simulink library "lib_astrodynamics"  (Simulink 7.7)
settings: Solver=ode45  StartTime=0.0  StopTime=10.0  RelTol=1e-3
libraries: lib_astrodynamics x4
settings Model: Creator=kkamiya  LastModifiedBy=yamaurashusaku

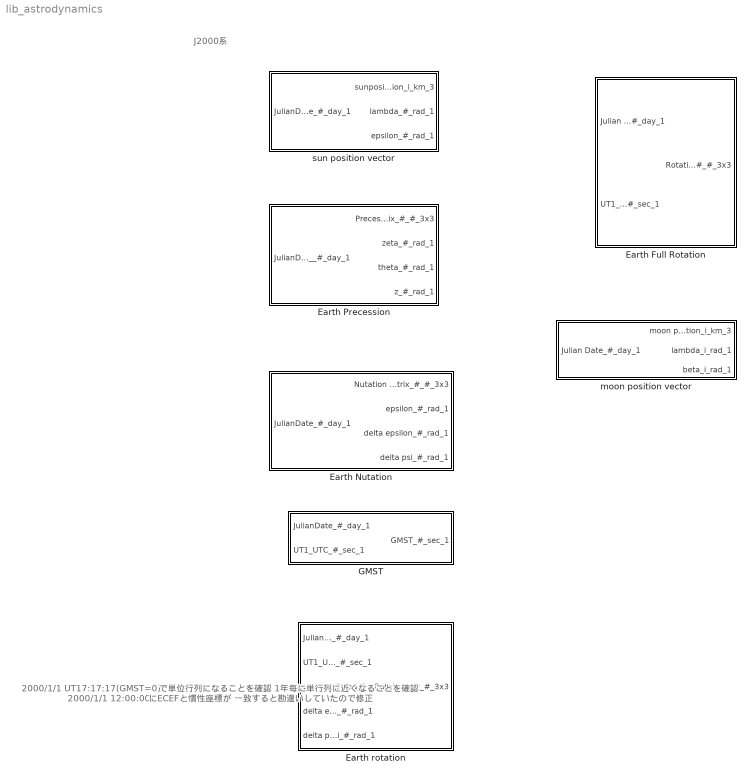
== system lib_astrodynamics ==
  note: J2000系
  note: 2000/1/1 UT17:17:17(GMST=0)で単位行列になることを確認
      | 1年毎に単行列に近くなることを確認
      | 2000/1/1 12:00:00にECEFと慣性座標が
      | 一致すると勘違いしていたので修正
  Earth Full Rotation : Subsystem
  Earth Nutation : Subsystem
  Earth Precession : Subsystem
  Earth rotation : Subsystem
  GMST : Subsystem
  moon position vector : Subsystem
  sun position vector : Subsystem

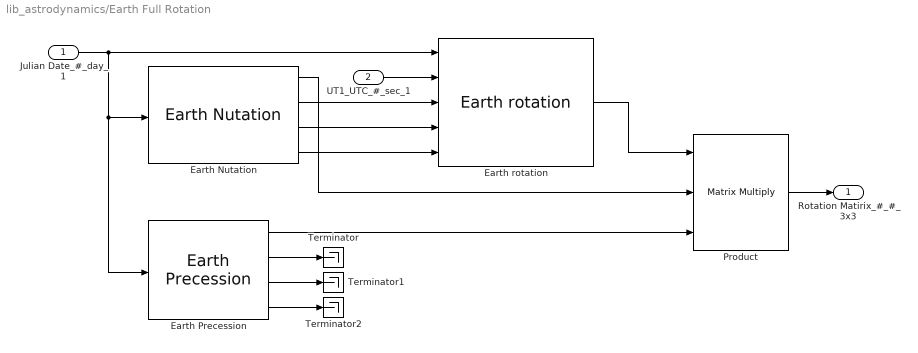
== system lib_astrodynamics/Earth Full Rotation ==
  Julian Date_#_day_1 : Inport
  UT1_UTC_#_sec_1 : Inport  Port=2
  Earth Nutation : lib_astrodynamics/Earth Nutation  SystemSampleTime=-1
  Earth Precession : lib_astrodynamics/Earth Precession  SystemSampleTime=-1
  Earth rotation : lib_astrodynamics/Earth rotation  SystemSampleTime=-1
  Product : Product  Inputs=3  Multiplication=Matrix(*)  RndMeth=Zero
  Terminator : Terminator
  Terminator1 : Terminator
  Terminator2 : Terminator
  Rotation Matirix_#_#_3x3 : Outport
  wires:
  Earth Nutation/2 -> Earth rotation/3
  Earth Nutation/3 -> Earth rotation/4
  Earth Nutation/4 -> Earth rotation/5
  Julian Date_#_day_1/1 -> Earth rotation/1, Earth Precession/1, Earth Nutation/1
  UT1_UTC_#_sec_1/1 -> Earth rotation/2
  Earth Precession/2 -> Terminator/1
  Earth Precession/3 -> Terminator1/1
  Earth Precession/4 -> Terminator2/1
  Earth Precession/1 -> Product/3
  Earth rotation/1 -> Product/1
  Earth Nutation/1 -> Product/2
  Product/1 -> Rotation Matirix_#_#_3x3/1

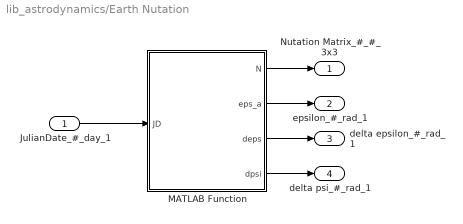
== system lib_astrodynamics/Earth Nutation ==
  JulianDate_#_day_1 : Inport
  MATLAB Function : Stateflow chart  TreatAsAtomicUnit=on
  Nutation Matrix_#_#_3x3 : Outport
  epsilon_#_rad_1 : Outport  Port=2
  delta epsilon_#_rad_1 : Outport  Port=3
  delta psi_#_rad_1 : Outport  Port=4
  wires:
  JulianDate_#_day_1/1 -> MATLAB Function/1(JD)
  MATLAB Function/1(N) -> Nutation Matrix_#_#_3x3/1
  MATLAB Function/2(eps_a) -> epsilon_#_rad_1/1
  MATLAB Function/3(deps) -> delta epsilon_#_rad_1/1
  MATLAB Function/4(dpsi) -> delta psi_#_rad_1/1

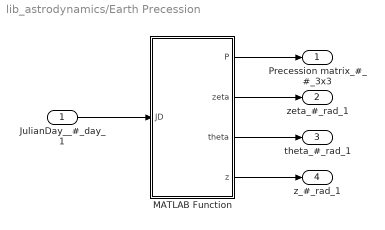
== system lib_astrodynamics/Earth Precession ==
  JulianDay__#_day_1 : Inport
  MATLAB Function : Stateflow chart  TreatAsAtomicUnit=on
  Precession matrix_#_#_3x3 : Outport
  zeta_#_rad_1 : Outport  Port=2
  theta_#_rad_1 : Outport  Port=3
  z_#_rad_1 : Outport  Port=4
  wires:
  JulianDay__#_day_1/1 -> MATLAB Function/1(JD)
  MATLAB Function/1(P) -> Precession matrix_#_#_3x3/1
  MATLAB Function/2(zeta) -> zeta_#_rad_1/1
  MATLAB Function/3(theta) -> theta_#_rad_1/1
  MATLAB Function/4(z) -> z_#_rad_1/1

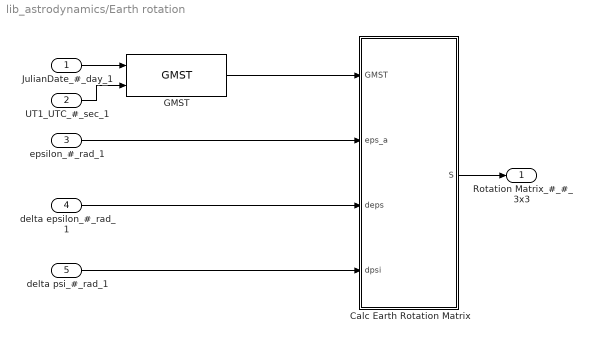
== system lib_astrodynamics/Earth rotation ==
  JulianDate_#_day_1 : Inport
  UT1_UTC_#_sec_1 : Inport  Port=2
  epsilon_#_rad_1 : Inport  Port=3
  delta epsilon_#_rad_1 : Inport  Port=4
  delta psi_#_rad_1 : Inport  Port=5
  Calc Earth Rotation Matrix : Stateflow chart  TreatAsAtomicUnit=on
  GMST : lib_astrodynamics/GMST
  Rotation Matrix_#_#_3x3 : Outport
  wires:
  JulianDate_#_day_1/1 -> GMST/1
  Calc Earth Rotation Matrix/1(S) -> Rotation Matrix_#_#_3x3/1
  delta psi_#_rad_1/1 -> Calc Earth Rotation Matrix/4(dpsi)
  delta epsilon_#_rad_1/1 -> Calc Earth Rotation Matrix/3(deps)
  epsilon_#_rad_1/1 -> Calc Earth Rotation Matrix/2(eps_a)
  GMST/1 -> Calc Earth Rotation Matrix/1(GMST)
  UT1_UTC_#_sec_1/1 -> GMST/2

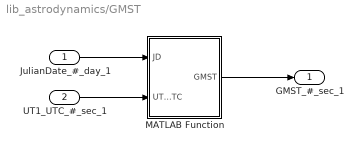
== system lib_astrodynamics/GMST ==
  JulianDate_#_day_1 : Inport
  UT1_UTC_#_sec_1 : Inport  Port=2
  MATLAB Function : Stateflow chart  TreatAsAtomicUnit=on
  GMST_#_sec_1 : Outport
  wires:
  JulianDate_#_day_1/1 -> MATLAB Function/1(JD)
  MATLAB Function/1(GMST) -> GMST_#_sec_1/1
  UT1_UTC_#_sec_1/1 -> MATLAB Function/2(UT1_UTC)

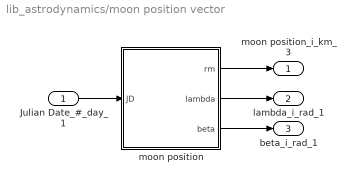
== system lib_astrodynamics/moon position vector ==
  Julian Date_#_day_1 : Inport
  moon position : Stateflow chart  TreatAsAtomicUnit=on
  moon position_i_km_3 : Outport
  lambda_i_rad_1 : Outport  Port=2
  beta_i_rad_1 : Outport  Port=3
  wires:
  moon position/1(rm) -> moon position_i_km_3/1
  Julian Date_#_day_1/1 -> moon position/1(JD)
  moon position/2(lambda) -> lambda_i_rad_1/1
  moon position/3(beta) -> beta_i_rad_1/1

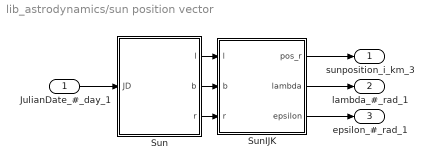
== system lib_astrodynamics/sun position vector ==
  JulianDate_#_day_1 : Inport
  Sun : Stateflow chart  TreatAsAtomicUnit=on
  SunIJK : Stateflow chart  TreatAsAtomicUnit=on
  sunposition_i_km_3 : Outport
  lambda_#_rad_1 : Outport  Port=2
  epsilon_#_rad_1 : Outport  Port=3
  wires:
  SunIJK/1(pos_r) -> sunposition_i_km_3/1
  SunIJK/2(lambda) -> lambda_#_rad_1/1
  SunIJK/3(epsilon) -> epsilon_#_rad_1/1
  Sun/1(l) -> SunIJK/1(l)
  Sun/2(b) -> SunIJK/2(b)
  Sun/3(r) -> SunIJK/3(r)
  JulianDate_#_day_1/1 -> Sun/1(JD)

== matlab function Earth Precession/MATLAB Function ==
  data: JD input double; P output double; zeta output double; theta output double; z output double
function [P,zeta,theta,z]= Precession(JD)

T = (JD - 2451545.0) / 36525.0;

SEC2RAD = pi / 180.0 / 3600.0;

T2 = T * T;
T3 = T2 * T;

zeta  = (2306.2181 * T + 0.30188 * T2 + 0.017998 * T3) * SEC2RAD;
theta = (2004.3109 * T - 0.42665 * T2 - 0.041833 * T3) * SEC2RAD;
z     = (2306.2181 * T + 1.09468 * T2 + 0.018203 * T3) * SEC2RAD;

P = RotationMatrix(3, -pi/2.0 - z) * RotationMatrix(1, theta) * RotationMatrix(3, pi/2.0 - zeta);

== matlab function sun position vector/SunIJK ==
  data: l input double; b input double; pos_r output double; r input double; lambda output double; epsilon output double
function [pos_r,lambda,epsilon]= fcn(l,b,r)
%#codegen
%   DESCRIPTION: Calculates Sun geocentric position from a given Julian day 
%                number, J2000
% 
%          (jd): Julian day number.(TDT)
%           (x): x position in J2000 [km]
%           (y): y position in J2000 [km]
%           (z): z position in J2000 [km]
epsilon = 23.43929111 * pi / 180.0;

sl = sin(l);

x = r * cos(l);
y = r * cos(epsilon) * sl;
z = r * sin(epsilon) * sl;
lambda = l;
  
pos_r=[x; y; z];

== matlab function Earth Nutation/MATLAB Function ==
  data: JD input double; N output double; eps_a output double; deps output double; dpsi output double
function [N, eps_a, deps, dpsi] = Nutation(JD)
%#codegen

SEC2RAD = pi / 180.0 / 3600.0;

T = (JD - 2451545.0) / 36525.0;
T2 = T * T;
T3 = T2 * T;

F   = ( 335778.877 + 1739527263.137 * T - 13.257 * T2 + 0.011 * T3 ) * SEC2RAD;
D   = (1072261.307 + 1602961601.328 * T -  6.891 * T2 + 0.019 * T3 ) * SEC2RAD;
Omg = ( 450160.280 -    6962890.539 * T +  7.455 * T2 + 0.008 * T3 ) * SEC2RAD;

eps_a = 84381.448 - 46.8150 * T - 0.00059 * T2 + 0.001813 * T3;

dpsi  = (-17.1996 - 0.01742 * T) * sin(Omg);
deps  = (  9.2025 + 0.00089 * T) * cos(Omg);

dpsi  = dpsi + ( 0.2062 + 0.00002 * T) * sin(2.0 * Omg);
deps  = deps + ( 0.5736 - 0.00031 * T) * cos(2.0 * (F-D+Omg));
dpsi  = dpsi + (-1.3187 - 0.00016 * T) * sin(2.0 * (F-D+Omg));

dpsi  = dpsi + (-0.2274 - 0.00002 * T) * sin(2.0 * (F+Omg));
deps  = deps + ( 0.0977 - 0.00005 * T) * cos(2.0 * (F+Omg));

eps_a = eps_a * SEC2RAD;
dpsi  = dpsi  * SEC2RAD;
deps  = deps  * SEC2RAD;

N = RotationMatrix(1, -eps_a-deps) * RotationMatrix(3, -dpsi) * RotationMatrix(1, eps_a);

== matlab function Earth rotation/Calc Earth Rotation Matrix ==
  data: GMST input double; S output double; eps_a input double; deps input double; dpsi input double
function S = fcn(GMST, eps_a, deps, dpsi)
%#codegen

GAST = GMST / 43200.0 * pi + dpsi * cos(eps_a + deps);

S = RotationMatrix(3, GAST);

== matlab function GMST/MATLAB Function ==
  data: JD input double; GMST output double; UT1_UTC input double
function GMST = GMST(JD, UT1_UTC)
%#codegen

MJD    = JD - 2400000.5 + UT1_UTC / 86400.0;
ut1_ss = (MJD - floor(MJD)) * 86400.0;
MJD     = floor(MJD);
T      = (MJD - 51544.5) / 36525.0;
T2 = T * T;

GMST   = 8640184.812866 * T;
% while GMST > 86400.0
%     GMST = GMST - 86400.0;
% end
%GMST   = fmod(8640184.812866 * T, 86400.0);
GMST   = GMST + (-6.2e-6 * T + 0.093104) * T2 + 24110.54841;
% while GMST > 86400.0
%     GMST = GMST - 86400.0;
% end
%GMST   = fmod(GMST, 86400.0);
% while GMST < 0.0
%     GMST = GMST + 86400.0;
% end

dsdmr  = 1.002737909350795 + 5.9006e-11 * T - 5.9e-15 * T2;

GMST   = GMST + dsdmr * ut1_ss;
%GMST    = fmod(cst, 86400.0);
% while GMST > 86400.0
%     GMST = GMST - 86400.0;
% end
% while GMST < 0.0
%     GMST = GMST + 86400.0;
% end
GMST = GMST - 86400.0 * floor(GMST / 86400.0);

== matlab function moon position vector/moon position ==
  data: JD input double; rm output double; lambda output double; beta output double
function [rm,lambda,beta] = moon_position(JD)
%#codegen

DEG2RAD = pi / 180.0;
SEC2RAD = pi / 180.0 / 3600.0;

T = (JD - 2451545.0) / 36525.0;
T2 = T * T;

L0 = (218.31617 + 481267.88088 * T - 1.3972 * T2) * DEG2RAD;
l  = (134.96292 + 477198.86753 * T              ) * DEG2RAD;
ld = (357.52543 +  35999.04944 * T              ) * DEG2RAD;
F  = ( 93.27283 + 483202.01873 * T              ) * DEG2RAD;
D  = (279.85027 + 445267.11135 * T              ) * DEG2RAD;

lambda = (L0 / SEC2RAD ...
       + 22640.0 * sin(l) ...
       +   769.0 * sin(2.0 * l) ...
       -  4586.0 * sin(l - 2.0 * D) ...
       +  2370.0 * sin(2.0 * D) ...
       -   668.0 * sin(ld) ...
       -   412.0 * sin(2.0 * F) ...
       -   212.0 * sin(2.0 * (l - D)) ...
       -   206.0 * sin(l + ld - 2.0 * D) ...
       +   192.0 * sin(l + 2.0 * D) ...
       -   165.0 * sin(ld - 2.0 * D) ...
       +   148.0 * sin(l - ld) ...
       -   125.0 * sin(D) ...
       -   110.0 * sin(l + ld) ...
       -    55.0 * sin(2.0 * (F - D))) * SEC2RAD;

beta   = (18520.0 * sin(F + lambda - L0 + (412.0 * sin(2.0 * F) + 541.0 * sin(l)) * SEC2RAD) ...
       -    526.0 * sin(F - 2.0 * D) ...
       +     44.0 * sin(l + F - 2.0 * D) ...
       -     31.0 * sin(-l + F - 2.0 * D) ...
       -     25.0 * sin(-2.0 * l + F) ...
       -     23.0 * sin(ld + F - 2.0 * D) ...
       +     21.0 * sin(-l + F) ...
       +     11.0 * sin(-ld + F - 2.0 * D)) * SEC2RAD;

r      = 385000.0 ...
       -  20905.0 * cos(l) ...
       -   3699.0 * cos(2.0 * D - l) ...
       -   2956.0 * cos(2.0 * D) ...
       -    570.0 * cos(2.0 * l) ...
       +    246.0 * cos(2.0 * (l - D)) ...
       -    205.0 * cos(ld - 2.0 * D) ...
       -    171.0 * cos(l + 2.0 * D) ...
       -    152.0 * cos(l + ld - 2.0 * D);

epsilon = 23.43929111 * DEG2RAD;

ce = cos(epsilon);
se = sin(epsilon);
cl = cos(lambda);
sl = sin(lambda);
cb = cos(beta);
sb = sin(beta);

x = r *                 cl * cb;
y = r * (ce * sl * cb - se * sb);
z = r * (se * sl * cb + ce * sb);

rm = [x; y; z];

== matlab function sun position vector/Sun ==
  data: JD input double; l output double; b output double; r output double
function [l,b,r] = fcn(JD)
%#codegen
%   DESCRIPTION: Calculates Moon geocentric longitude, latitude, and
%                distance for a given Julian day number, J2000 ecliptic
% 
%          (jd): Julian day number.(TDT)
%           (l): Receives Sun geocentric longitude, in radians.
%           (b): Receives Sun geocentric latitude, in radians. = 0
%           (r): Receives Sun geocentric distance, in km.
DEG2RAD = pi / 180.0;

T = (JD - 2451545.0) / 36525.0;
	
M = (357.5256 + 35999.045 * T) * DEG2RAD;
l = (282.94 + (6892.0 * sin(M) + 72.0 * sin(2.0 * M) + 1250.09115 * T) / 3600.0 - 0.002652) * DEG2RAD + M;
b = 0.0;
r = 149619000.0 - 2499000.0 * cos(M) - 21000.0 * cos(2.0 * M);
